simulink model "GenMapped"  (R2021b)
settings: Solver=VariableStepAuto  StartTime=0.0  StopTime=inf  RelTol=1e-3  EnableMultiTasking=on
model workspace (MAT data in the model file):
  EV_current = 200
  EV_motion = [20 4 0.8]
  EV_sf = 2000
  Fs = 0
  Fv = 0.0025
  Jcomp = 0.0227
  Ki = 251.3274
  Kisa = 346.6583
  Kp_d = 0.47149
  Kp_q = 0.52125
  Ksa = 85.4316
  Ksf = 1996.2651
  Ld = 0.0003752
  Ldq = [0.0003752 0.0004148]
  Lq = 0.0004148
  Mechanical = [0.0227 0.0025 0]
  P = 4
  PolePairs = 4
  Rs = 0.2
  T_max = 120
  T_mtpa = [0 13.3131834767 26.6278836885 39.9456159322 53.2678926341 66.5962219318 79.9321062746 93.277041051 106.632513247 120.000000141]
  ba = 3.4029
  gen.max_trq = 247.580645161
  gen.max_pwr = 102.101761242
  gen.spd = [0 500 1000 1500 2000 2500 3000 3500 3938.11074919 4000 4500 5000 5500 6000 6500 7000 7500 8000 8500 9000 9500 10000 10500 11000 11500 12000 12500]
  gen.trq = [247.580645161 247.580645161 247.580645161 247.580645161 247.580645161 247.580645161 247.580645161 247.580645161 247.580645161 243.75 216.666666667 195 177.272727273 162.5 150 139.285714286 130 121.875 114.705882353 108.333333333 102.631578947 97.5 92.8571428571 88.6363636364 84.7826086957 81.25 78]
  gen.trq_cp = [243.75 216.666666667 195 177.272727273 162.5 150 139.285714286 130 121.875 114.705882353 108.333333333 102.631578947 97.5 92.8571428571 88.6363636364 84.7826086957 81.25 78]
  gen.J = 0.02
  gen.damp = 0.001
  gen.Tc = 0.02
  gen.map.spdindex = [0 1000 2000 3000 3857 4000 5000 6000 7000 8000 9000 10000 11000 12000 12584]
  gen.map.trqindex = [10 25 50 75 100 125 150 175 200 225 235.201612903]
  gen.map.eff = [84  90  90  90  90  90  90  90  90  90  90  90  90  90  90; 84  90  93  95  95  95  96  95  95  95  95  93  93  93  93; 84  90  93  95  95  95  96  95  96  95  95  95  95  93  93; 84  90  93  95  95  95  96  96  96  95  95  93  95  93  93; 84  90  93  95  95  95  96  96  96  95  95  93  93  93  93; 84  88  90  93  93  95  95  96  95  93  93  93  93  93  93; 84  88  90  90  90  93  95  95  93  93  93  93  93  93  93; 84  88  90  90  90  90  93  93  93  93  93  93  93  93  93; 84  84  88  90  90  90  90  93  93  93  93  93  93  93  93; 84  84  88  90  90  90  90  93  93  93  93  93  93  93  93; 84  84  88  90  90  90  90  93  93  93  93  93  93  93  93]
  gen.m = 20
  gen.Cp = 200
  id_mtpa = [0 -0.114523352646 -0.457989076459 -1.03008464374 -1.83029075221 -2.85788367342 -4.11193850568 -5.59133329791 -7.29475400168 -9.22070020138]
  idq0 = [0 0]
  idq_limits = [-9.220699542 166.993501392 167.247872355]
  iq_mtpa = [0 18.5827440345 37.1633719111 55.7397734896 74.3098506185 92.871523015 111.422734008 129.961456105 148.485696337 166.993501356]
  lambda_pm = 0.1194
  mechanical = [0.0227 0.0025 0]
  omega_init = 0
  theta_init = 0
libraries: autolibmappedmotor x1
settings Model: DataDictionary=GenMapped.sldd  ModifiedByFormat=The MathWorks, Inc.  SimulationMode=accelerator  PauseTimes=10  Creator=The MathWorks, Inc.  LastModifiedBy=The MathWorks, Inc.
settings SolverCC: AlgebraicLoopSolver=TrustRegion  DecoupledContinuousIntegration=on
settings DataIOCC: DSMLogging=off  ReturnWorkspaceOutputs=off
settings DebuggingCC: SFMachineParentedDataDiag=warning  ArithmeticOperatorsInVariantConditions=warning
settings ModelReferenceCC: PropagateSignalLabelsOutOfModel=off
settings SFSimCC: SimUseLocalCustomCode=off  CustomCodeUndefinedFunction=UseInterfaceOnly
settings RTWCC: RTWUseLocalCustomCode=off
settings CodeAppCC: StateflowObjectComments=on
settings GRTTargetCC: TargetLangStandard=C89/C90 (ANSI)
settings ConfigComp: CovMetricSettings=dsw  CovSaveCumulativeToWorkspaceVar=on  CovSaveSingleToWorkspaceVar=on  CovExternalEMLEnable=off
settings SimscapeCC: SimscapeNormalizeSystem=off  SimscapeNominalValues={1, 'bar'; 1, 'cm^3/s'; 1, 'bar*kg/s'; 1, 'kJ/kg'; 1, 'kW'; }

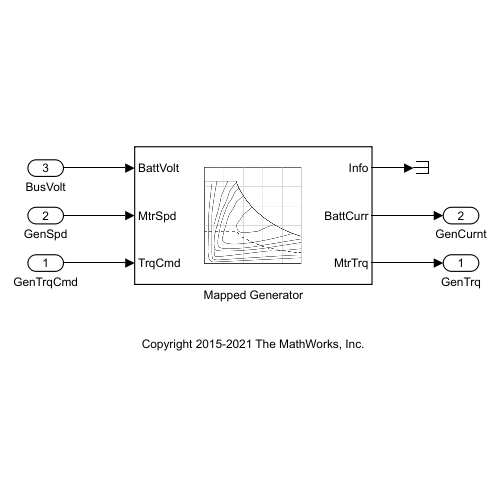
[thumbnail: Simulink's stored preview of the top-level diagram]
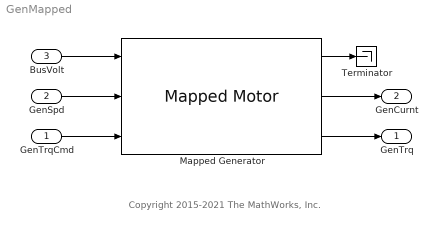
== system GenMapped ==
  note: Copyright 2015-2021 The MathWorks, Inc.
  GenTrqCmd : Inport
  GenSpd : Inport  Port=2
  BusVolt : Inport  Port=3
  Mapped Generator : autolibmappedmotor/Mapped Motor  port_config=Speed  param_by=Maximum torque and power  w_t=[ 0 375 750 800 ]  T_t=[0.09 0.08 0.07 0]  torque_max=247.5806  power_max=102.1e3  Tc=0.02  param_loss=Tabulated efficiency data  eff=100  w_eff=375  T_eff=0.08  Piron=0  Pbase=0  w_eff_bp=gen.map.spdindex.*pi/30  T_eff_bp=gen.map.trqindex  Temp_eff_bp=[233.15 293.15 373.15]  losses_table=[1 2;3 4]  losses_table_3d=cat(3,[1.49 1.67 2.21 3.10; 0.42 0.69 1.14 2.03; 0.06 0.24 0.78 1.68; 0.42 0.69 1.14 2.03; 1.49 1.67 2.21 3.10],[1.49 1.67 2.21 3.10; 0.42 0.69 1.14 2.03; 0.06 0.24 0.78 1.68; 0.42 0.69 1.14 2.03; 1.49 1.67 2.21 3.10],[1.49 1.67 2.21 3.10; 0.42 0.69 1.14 2.03; 0.06 0.24 0.78 1.68; 0.42 0.69 1.14 2.03; 1.49 1.67 2.21 3.10])  efficiency_table=gen.map.eff'  efficiency_table_3d=cat(3,[95 95 95 95; 95 95 95 95; 95 95 95 95; 95 95 95 95; 95 95 95 95],[95 95 95 95; 95 95 95 95; 95 95 95 95; 95 95 95 95; 95 95 95 95],[95 95 95 95; 95 95 95 95; 95 95 95 95; 95 95 95 95; 95 95 95 95])  J=5e-6  b=1e-5  omega_o=0  T_t_extended=[0 0.07 0.08 0.09 0.08 0.07 0]  w_t_extended=[-800 -750 -375 0 375 750 800]  KLossIron=0  KLossCopper=0  x_w_eff_vec=[-1317.7933984258 -1256.63706143592 -1151.91730631626 -1047.1975511966 -942.477796076938 -837.758040957278 -733.038285837618 -628.318530717959 -523.598775598299 -418.879020478639 -403.904095496528 -314.159265358979 -209.43951023932 -104.71975511966 0 104.71975511966 209.43951023932 314.159265358979 403.904095496528 418.879020478639 523.598775598299 628.318530717959 733.038285837618 837.758040957278 942.477796076938 1047.1975511966 1151.91730631626 1256.63706143592 1317.7933984258]  x_T_eff_vec=[-235.201612903226 -225 -200 -175 -150 -125 -100 -75 -50 -25 -10 10 25 50 75 100 125 150 175 200 225 235.201612903226]  x_tmp_eff_vec=[-0.09 -0.06 -0.03 0 0.03 0.06 0.09]  x_losses_mat=[23329.3540804387 22317.4688443079 19837.7500838292 17358.0313233506 14878.3125628719 12398.5938023933 9918.8750419146 7439.15628143595 4959.4375209573 2479.71876047865 1464.21488713978 1317.7933984258 2306.13844724515 4612.27689449029 6918.41534173544 9224.55378898058 11530.6922362257 13836.8306834709 16142.969130716 18449.1075779612 20755.2460252063 21696.299294808;22246.6822127514 21281.7566856083 18917.117053874 16552.4774221398 14187.8377904055 11823.1981586713 9458.558526937 7093.91889520275 4729.2792634685 2364.63963173425 1396.26340159546 1256.63706143592 2199.11485751285 4398.22971502571 6597.34457253856 8796.45943005141 10995.5742875643 13194.6891450771 15393.80400259 17592.9188601028 19792.0337176157 20689.4144578588;20392.7920283555 19508.2769618076 17340.6906327178 15173.1043036281 13005.5179745384 10837.9316454486 8670.34531635892 4547.0419986168 3031.3613324112 2167.58632908973 1279.90811812918 1151.91730631626 2015.85528605345 2879.79326579064 4319.68989868596 8063.4211442138 10079.2764302672 12095.1317163207 14110.9870023741 16126.8422884276 18142.697574481 18965.2965863706;18538.9018439595 17734.7972380069 15764.2642115617 13793.7311851165 11823.1981586713 9852.66513222605 7882.13210578084 5911.59907933563 2755.78302946473 1970.53302644521 1163.55283466289 1047.1975511966 1832.59571459404 2617.99387799149 5497.78714378213 7330.38285837618 9162.97857297022 10995.5742875643 12828.1700021583 14660.7657167524 16493.3614313464 17241.1787148824;16685.0116595636 15961.3175142062 14187.8377904055 12414.3580666048 10640.8783428041 8867.39861900344 4960.40945303651 3720.30708977738 2480.20472651826 1240.10236325913 1047.1975511966 942.477796076938 1178.09724509617 2356.19449019234 3534.29173528851 4712.38898038468 8246.6807156732 9896.01685880784 11545.3530019425 13194.6891450771 14844.0252882118 15517.0608433941;14831.1214751676 14187.8377904055 12611.4113692493 11034.9849480932 9458.558526937 7882.13210578084 4409.25284714356 3306.93963535767 2204.62642357178 1102.31321178589 930.842267730309 837.758040957278 1047.1975511966 2094.39510239319 3141.59265358979 4188.79020478639 7330.38285837618 8796.45943005141 10262.5360017266 11728.6125734019 13194.6891450771 13792.9429719059;12977.2312907717 12414.3580666048 11034.9849480932 9655.61182958152 8276.23871106988 4822.62030156327 3054.32619099008 2290.74464324256 1527.16309549504 964.524060312655 814.486984264021 733.038285837618 916.297857297022 1466.07657167524 2199.11485751286 2932.15314335048 4581.48928648511 7696.90200129499 8979.71900151082 10262.5360017266 11545.3530019425 12068.8251004177;11123.3411063757 10640.8783428041 9458.558526937 8276.23871106988 4960.40945303651 3272.49234748937 2617.9938779915 1963.49540849362 1653.46981767884 826.734908839418 698.131700797732 628.318530717959 785.398163397447 1570.79632679489 1884.95559215388 2513.27412287184 3141.5926535898 4712.38898038468 7696.90200129499 8796.45943005141 9896.01685880784 10344.7072289294;13683.4751705416 13089.9693899575 11635.5283466289 6896.86559255823 4133.67454419709 3444.72878683091 2181.66156499292 1636.24617374469 1090.83078249646 545.415391248229 581.776417331443 523.598775598299 523.598775598299 1047.1975511966 1570.7963267949 2094.3951023932 3272.49234748936 3926.99081698724 6414.08500107916 10471.975511966 11780.9724509617 12315.1276534874;10946.7801364333 10471.975511966 9308.4226773031 8144.86984264021 4729.2792634685 2755.78302946473 2204.62642357178 1653.46981767884 1102.31321178589 551.156605892946 465.421133865155 418.879020478639 523.598775598298 1047.1975511966 1570.79632679489 2094.39510239319 2617.99387799149 4398.22971502571 7330.38285837618 8377.58040957278 9424.77796076938 9852.10212278992;10555.4327465558 10097.6023874132 8975.64656658951 7853.69074576582 6731.73492494213 3800.17294149958 2125.81102892909 1594.35827169682 1062.90551446455 531.452757232273 448.782328329475 403.904095496528 504.880119370659 1009.76023874132 1514.64035811198 2019.52047748264 3534.16083559461 ...(+6444 chars)]  x_losses_mat_3d=[37.8947368421052 25.2631578947368 12.6315789473684 0 12 24 36;18.9473684210526 12.6315789473684 6.3157894736842 0 5.99999999999999 12 18;0 0 0 0 0 0 0;18 12 5.99999999999999 0 6.3157894736842 12.6315789473684 18.9473684210526;36 24 12 0 12.6315789473684 25.2631578947368 37.8947368421052]  CalLossMapData={}  CalLossWithTempMapData={}  aMode=1  RefBlkName='autolibmappedmotor/Mapped Motor'
      settings: SourceProductBaseCode=PW,DR,MT,UV,VE
  Terminator : Terminator
  GenTrq : Outport  VectorParamsAs1DForOutWhenUnconnected=off
  GenCurnt : Outport  Port=2  VectorParamsAs1DForOutWhenUnconnected=off
  wires:
  GenTrqCmd/1 -> Mapped Generator/3
  GenSpd/1 -> Mapped Generator/2
  BusVolt/1 -> Mapped Generator/1
  Mapped Generator/2 -> GenCurnt/1
  Mapped Generator/3 -> GenTrq/1
  Mapped Generator/1 -> Terminator/1
